simulink model "torqueBalancing2012b"  (Simulink 8.0)
settings: Solver=FixedStepDiscrete  StartTime=0.0  StopTime=CONFIG.SIMULATION_TIME  FixedStep=CONFIG.Ts  RelTol=1e-3
InitFcn:
  | initTorqueBalancing;
values from neighbouring files (symbols this model uses):
  baseToWorldRotationPort = ['/' WBT_modelName '/floatingBaseRotationMatrix:i']    [initTorqueBalancing.m]
  WBT_modelName = 'matlabTorqueBalancing'    [initTorqueBalancing.m]
undefined symbols (not defined in the file or in its folder): bVectorConstraints, CONFIG, ConstraintsMatrix, DiscIntNeverNeededParam, gain, impedencesSat, reg, ROBOT_DOF, ROBOT_DOF_FOR_SIMULINK, sat, SM, sm, Ts
libraries: WBToolboxLibrary x139, simulink x11, WBCLibrary x2
(part 3 of 3)

== matlab function DesValues/State Machine/nu/MATLAB Function ==
  data: JcLeftFoot input double; JcRightFoot input double; activeFeetConstraints input double; y output double; qD input double; reg parameter double
function y = fcn(JcLeftFoot,JcRightFoot,activeFeetConstraints,qD,reg)
%#codegen

Jc = [activeFeetConstraints(1)*JcLeftFoot;
      activeFeetConstraints(2)*JcRightFoot];

pinvJb = (Jc(:,1:6)'*Jc(:,1:6) + reg.pinvDampVb*eye(6))\Jc(:,1:6)';  
  
% pinvJb = pinv(Jc(:,1:6));

y = -pinvJb*Jc(:,7:end)*qD;

== matlab function DesValues/State Machine/stateMachineFCN ==
  data: wrench_rightFoot input double; wrench_leftFoot input double; w_H_b output double; CoMDes output double; qDes output double; constraints output double; state data_store_memory double; CoM_0 input double; q0 input double; l_sole_CoM input double; r_sole_CoM input double; qj input double; t input double; l_sole_H_b input double; r_sole_H_b input double; tSwitch data_store_memory double; sm parameter double; impedances output double; gain parameter double; currentState output double; w_H_r_sole_switch data_store_memory double
function [w_H_b, CoMDes,qDes,constraints,impedances,currentState] = ...
    stateMachineFCN(wrench_rightFoot,wrench_leftFoot,CoM_0, q0, l_sole_CoM,r_sole_CoM,qj, t, l_sole_H_b, r_sole_H_b, sm,gain)
%#codegen
 
[CoMDes,qDes,constraints, currentState,impedances,w_H_b] = ...
    stateMachine(CoM_0, q0, l_sole_CoM,r_sole_CoM,qj, t, wrench_rightFoot,wrench_leftFoot,l_sole_H_b, r_sole_H_b, sm,gain);

== matlab function DesValues/nonlinearImpedances/nonlinearPosturalGains  ==
  data: qDes input double; nonlinearImpedences output double; q input double; qMin input double; qMax input double; gain parameter double
function nonlinearImpedences = fcn(qDes,q,qMin,qMax,gain)
    %#codegen
    impedences_at_0     = gain.impedances;
    increasingRatesImp  = (gain.increasingRatesImp)';
    qTildeMax           = gain.qTildeMax;

    tp =  pi./(2*(qMax-qDes));
    tn = -pi./(2*(qMin-qDes));

    
    qTilde = q - qDes;
            
    nonlinearImpedences = (impedences_at_0'   + increasingRatesImp.*tan(pi.*qTilde./(2*qTildeMax)).^2)';
%                                                increasingRatesImp.*tan((tp.*stepFcn(qTilde) + tn.*stepFcn(-qTilde)).*qTilde).^2)';
                                           
end

function y = stepFcn(x) 
   %#codegen
   y = x > 0; 
end

== matlab function Dump and visualize/plotNorms/norm ==
  data: u input double; normU output double
function normU = fcn(u)
%#codegen

normU = norm(u);

== matlab function Dump and visualize/plotNorms/norm1 ==
  data: u input double; normU output double
function normU = fcn(u)
%#codegen

normU = norm(u);

== matlab function controller_QP/tau(f)  ==
  data: tauModel output double; Sigma output double; NA output double; fHdotDesC1C2 output double; HessianMatrixQP1Foot output double; gradientQP1Foot output double; ConstraintsMatrixQP1Foot output double; bVectorConstraintsQp1Foot output double; HessianMatrixQP2Feet output double; gradientQP2Feet output double; ConstraintsMatrixQP2Feet output double; bVectorConstraintsQp2Feet output double; constraints input double; ROBOT_DOF_FOR_SIMULINK input double; ConstraintsMatrix input double; bVectorConstraints input double; q input double; qDes input double; v input double; M input double; h input double; H input double; w_H_l_sole input double; w_H_r_sole input double; JL input double; JR input double; dJLv input double; dJRv input double; xcom input double; J_CoM input double; desired_x_dx_ddx_CoM input double; impedances input double; intErrorCoM input double; ki_int_qtilde input double; reg parameter double; gain parameter double; errorCoM output double; qTilde output double; f output double; Deltaphi input double
function [tauModel,Sigma,NA,fHdotDesC1C2, ...
          HessianMatrixQP1Foot,gradientQP1Foot,ConstraintsMatrixQP1Foot,bVectorConstraintsQp1Foot,...
          HessianMatrixQP2Feet,gradientQP2Feet,ConstraintsMatrixQP2Feet,bVectorConstraintsQp2Feet,...
          errorCoM,qTilde,f]    =  ...
          controllerFCN(constraints,ROBOT_DOF_FOR_SIMULINK,ConstraintsMatrix,bVectorConstraints,...
          q,qDes,v, M, h , H,w_H_l_sole, w_H_r_sole, JL,JR, dJLv,dJRv, xcom,J_CoM, desired_x_dx_ddx_CoM,...
          impedances, intErrorCoM,ki_int_qtilde,reg,gain,Deltaphi)
%#codegen
pos_leftFoot   = w_H_l_sole(1:3,4);
rotMatLeftFoot = w_H_l_sole(1:3,1:3);

pos_rightFoot   = w_H_r_sole(1:3,4);
rotMatRightFoot = w_H_r_sole(1:3,1:3);

footSize       = gain.footSize;
gainsPCOM      = gain.PCOM;
gainsICOM      = gain.ICOM;
gainsDCOM      = gain.DCOM;
DgainMomentum  = gain.DAngularMomentum;
PgainMomentum  = gain.PAngularMomentum;
dampings       = gain.dampings;

e1              = [1;0;0];
e2              = [0;1;0];
e3              = [0;0;1]; 
ROBOT_DOF       = size(ROBOT_DOF_FOR_SIMULINK,1);


gravAcc         = 9.81;
m               = M(1,1);
Mb              = M(1:6,1:6);
Mbj             = M(1:6,7:end);
% Mj              = M(7:end,7:end);

St              = [  zeros(6,ROBOT_DOF);
                   eye(ROBOT_DOF,ROBOT_DOF)];
grav            = [ zeros(2,1);
                   -m*gravAcc;
                    zeros(3,1)];
                



xDcom           = J_CoM(1:3,:)*v;
qD              = v(7:end);
xDDcomStar      = desired_x_dx_ddx_CoM(:,3) - gainsPCOM*(xcom - desired_x_dx_ddx_CoM(:,1)) - gainsICOM*intErrorCoM - gainsDCOM*(xDcom - desired_x_dx_ddx_CoM(:,2));
Pr              = pos_rightFoot - xcom; % Application point of the contact force on the right foot w.r.t. CoM
Pl              = pos_leftFoot  - xcom; % Application point of the contact force on the left foot w.r.t. CoM


AL = [ eye(3),   zeros(3);
       Sf(Pl),  eye(3)];
AR = [ eye(3), zeros(3);
        Sf(Pr), eye(3) ];
    
A    = [ AL, AR];

Jc   = [ JL*constraints(1) ;
         JR*constraints(2)];
JcDv = [ dJLv*constraints(1) ;
         dJRv*constraints(2)];

JcMinv          = Jc/M;
JcMinvSt        = JcMinv*St;
JcMinvJct       = JcMinv*transpose(Jc);

pinvA         = pinv( A, reg.pinvTol)*constraints(1)*constraints(2) + [inv(AL);zeros(6)]*constraints(1)*(1-constraints(2)) + [zeros(6);inv(AR)]*constraints(2)*(1-constraints(1)); 
% PInv_JcMinvSt = pinv( JcMinvSt, PINV_TOL);
PInv_JcMinvSt = JcMinvSt'/(JcMinvSt*JcMinvSt' + reg.pinvDamp*eye(size(JcMinvSt,1)));
  
% linear approssimation of centroidal orientation
qTilde           =  q-qDes;

HDotDes  = [ m*xDDcomStar ;
            -DgainMomentum*H(4:end)-PgainMomentum*Deltaphi]; 
         
%%%%
        
NL        = eye(ROBOT_DOF) - PInv_JcMinvSt*JcMinvSt;

f_HDot           = pinvA*(HDotDes - grav);

fHdotDesC1C2     =  f_HDot*constraints(1)*constraints(2);

NA               = (eye(12,12)-pinvA*A)*constraints(1)*constraints(2);
JBar             = transpose(Jc(:,7:end)) - Mbj'/Mb*transpose(Jc(:,1:6)); % multiplier of f in tau0

Sigma            = -(PInv_JcMinvSt*JcMinvJct + NL*JBar);
SigmaNA          = Sigma*NA;

tauModel         = PInv_JcMinvSt*(JcMinv*h - JcDv) + NL*(h(7:end) - Mbj'/Mb*h(1:6) - diag(impedances)*qTilde  -ki_int_qtilde -diag(dampings)*NL*qD);

CL               = ConstraintsMatrix; 
CL(end-4,1:3)    = -e3'*rotMatLeftFoot;                
CL(end-3,:)      = [ footSize(1,1)*e3'*rotMatLeftFoot', e2'*rotMatLeftFoot'];
CL(end-2,:)      = [-footSize(1,2)*e3'*rotMatLeftFoot',-e2'*rotMatLeftFoot'];

CL(end-1,:)      = [ footSize(2,1)*e3'*rotMatLeftFoot',-e1'*rotMatLeftFoot'];
CL(end  ,:)      = [-footSize(2,2)*e3'*rotMatLeftFoot', e1'*rotMatLeftFoot'];

CR               = ConstraintsMatrix;
CR(end-4,1:3)    = -e3'*rotMatRightFoot;  
CR(end-3,:)      = [ footSize(1,1)*e3'*rotMatRightFoot', e2'*rotMatRightFoot'];
CR(end-2,:)      = [-footSize(1,2)*e3'*rotMatRightFoot',-e2'*rotMatRightFoot'];

CR(end-1,:)      = [ footSize(2,1)*e3'*rotMatRightFoot',-e1'*rotMatRightFoot'];
CR(end  ,:)      = [-footSize(2,2)*e3'*rotMatRightFoot', e1'*rotMatRightFoot'];


ConstraintsMatrix2Feet    = blkdiag(CL,CR);
bVectorConstraints2Feet   = [bVectorConstraints;bVectorConstraints];

ConstraintsMatrixQP1Foot  = constraints(1) * (1 - constraints(2)) * CL + ...
                           constraints(2) * (1 - constraints(1)) * CR;
bVectorConstraintsQp1Foot = bVectorConstraints;

ConstraintsMatrixQP2Feet  = ConstraintsMatrix2Feet*NA;
bVectorConstraintsQp2Feet = bVectorConstraints2Feet-ConstraintsMatrix2Feet*f_HDot;

HessianMatrixQP2Feet      = SigmaNA'*SigmaNA + eye(size(SigmaNA,2))*reg.HessianQP;
gradientQP2Feet           = SigmaNA'*(tauModel + Sigma*f_HDot);

A1Foot                    = AL*constraints(1)*(1-constraints(2)) + AR*constraints(2)*(1-constraints(1));
HessianMatrixQP1Foot      = A1Foot'*A1Foot + eye(size(A1Foot,2))*reg.HessianQP;
gradientQP1Foot           = -A1Foot'*(HDotDes - grav);

f0                        = -pinv(SigmaNA, reg.pinvTol)*(tauModel + Sigma*f_HDot);

f                         = f_HDot + NA*f0;

errorCoM = xcom - desired_x_dx_ddx_CoM(:,1);

== matlab function emergency stop: joint limits/MATLAB Function ==
  data: umin input double; umax input double; u input double; inRange output double; tol input double
function inRange = checkRange(umin, umax, u, tol)
%#codegen

res = u < umin + tol | u > umax - tol;
res = sum(res);
if res==0
    inRange = 1;
else
    inRange = 0;
    u < umin + tol | u > umax - tol
end

== matlab function DesValues/State Machine Walking/w_H_root_link3/fromImuToHomogeousTransformFCN ==
  data: imu_H_link input double; imu_H_link_0 input double; link_H_root input double; inertial_0 input double; inertial input double; w_H_root output double; CONFIG parameter double
function w_H_root = fromBaseToWorldWithImuFCN(imu_H_link,imu_H_link_0,link_H_root,inertial_0,inertial,CONFIG)
%#codegen
w_H_root = fromBaseToWorldWithImu(imu_H_link,imu_H_link_0,link_H_root,inertial_0,inertial,CONFIG);

== matlab function DesValues/centroidalOrient_partialDer/Jw0_base/Generate_Jw0base/MATLAB Function ==
  data: vb1 output double; vb2 output double; vb3 output double; vb4 output double; vb5 output double; vb6 output double
function [vb1,vb2, vb3, vb4, vb5, vb6] = gen_vb()
%#codegen

vb1 = [1;0;0;0;0;0];
vb2 = [0;1;0;0;0;0];
vb3 = [0;0;1;0;0;0];
vb4 = [0;0;0;1;0;0];
vb5 = [0;0;0;0;1;0];
vb6 = [0;0;0;0;0;1];

end

== matlab function DesValues/centroidalOrient_partialDer/Jw0_base/Generate_Jw0base/MATLAB Function1 ==
  data: H1 input double; Jw0b output double; H2 input double; H3 input double; H4 input double; H5 input double; H6 input double
function Jw0b = reorder_Jwb(H1,H2,H3,H4,H5,H6)
%#codegen

Jw0b = [H1 H2 H3 H4 H5 H6];

end

== matlab function DesValues/centroidalOrient_partialDer/Jc0/MATLAB Function ==
  data: Jclf input double; Jc0 output double; Jcrf input double
function Jc0 = fcn(Jclf,Jcrf)
%#codegen

Jc0 = [Jclf;Jcrf];

end

== matlab function DesValues/centroidalOrient_partialDer/Jw0_joints/Generate_Jw0torso/MATLAB Function ==
  data: dqj1 output double; dqj2 output double; dqj3 output double
function [dqj1,dqj2,dqj3] = gen_vb()
%#codegen
ndof = 23;

dqj1 = zeros(ndof,1);
dqj2 = zeros(ndof,1);
dqj3 = zeros(ndof,1);

dqj1(1) = 1;
dqj2(2) = 1;
dqj3(3) = 1;

end

== matlab function DesValues/centroidalOrient_partialDer/Jw0_joints/Generate_Jw0torso/MATLAB Function1 ==
  data: H1 input double; Jw0j1 output double; H2 input double; H3 input double
function Jw0j1 = reorder_Jwj(H1,H2,H3)
%#codegen

Jw0j1 = [H1 H2 H3];

end

== matlab function DesValues/centroidalOrient_partialDer/Jw0_joints/Generate_Jw0Rarm/MATLAB Function ==
  data: dqj9 output double; dqj10 output double; dqj11 output double; dqj12 output double; dqj13 output double
function [dqj9,dqj10, dqj11, dqj12, dqj13] = gen_vb()
%#codegen
ndof = 23;

dqj9  = zeros(ndof,1);
dqj10 = dqj9;
dqj11 = dqj10;
dqj12 = dqj11;
dqj13 = dqj12;

dqj9(9)  = 1;
dqj10(10) = 1;
dqj11(11) = 1;
dqj12(12) = 1;
dqj13(13) = 1;

end

== matlab function DesValues/centroidalOrient_partialDer/Jw0_joints/Generate_Jw0Rarm/MATLAB Function1 ==
  data: H1 input double; Jw0j3 output double; H2 input double; H3 input double; H4 input double; H5 input double
function Jw0j3 = reorder_Jwj(H1,H2,H3,H4,H5)
%#codegen

Jw0j3 = [H1 H2 H3 H4 H5];

end

== matlab function DesValues/centroidalOrient_partialDer/Jw0_joints/Generate_Jw0Lleg/MATLAB Function ==
  data: dqj14 output double; dqj15 output double; dqj16 output double; dqj17 output double; dqj18 output double
function [dqj14,dqj15, dqj16, dqj17, dqj18] = gen_vb()
%#codegen
ndof = 23;

dqj14 = zeros(ndof,1);
dqj15 = dqj14;
dqj16 = dqj15;
dqj17 = dqj16;
dqj18 = dqj17;

dqj14(14) = 1;
dqj15(15) = 1;
dqj16(16) = 1;
dqj17(17) = 1;
dqj18(18) = 1;

end

== matlab function DesValues/centroidalOrient_partialDer/Jw0_joints/Generate_Jw0Lleg/MATLAB Function1 ==
  data: H1 input double; Jw0j4 output double; H2 input double; H3 input double; H4 input double; H5 input double
function Jw0j4 = reorder_Jwj(H1,H2,H3,H4,H5)
%#codegen

Jw0j4 = [H1 H2 H3 H4 H5];

end

== matlab function DesValues/centroidalOrient_partialDer/Jw0_joints/Generate_Jw0Rleg/MATLAB Function ==
  data: dqj19 output double; dqj20 output double; dqj21 output double; dqj22 output double; dqj23 output double
function [dqj19,dqj20, dqj21, dqj22, dqj23] = gen_vb()
%#codegen
ndof = 23;

dqj19 = zeros(ndof,1);
dqj20 = dqj19;
dqj21 = dqj20;
dqj22 = dqj21;
dqj23 = dqj22;

dqj19(19) = 1;
dqj20(20) = 1;
dqj21(21) = 1;
dqj22(22) = 1;
dqj23(23) = 1;

end

== matlab function DesValues/centroidalOrient_partialDer/Jw0_joints/Generate_Jw0Rleg/MATLAB Function1 ==
  data: H1 input double; Jw0j5 output double; H2 input double; H3 input double; H4 input double; H5 input double
function Jw0j5 = reorder_Jwj(H1,H2,H3,H4,H5)
%#codegen

Jw0j5 = [H1 H2 H3 H4 H5];

end

== matlab function DesValues/centroidalOrient_partialDer/Jw0_joints/MATLAB Function ==
  data: Jw01 input double; Jw0j output double; Jw02 input double; Jw03 input double; Jw04 input double; Jw05 input double
function Jw0j = fcn(Jw01,Jw02,Jw03,Jw04,Jw05)
%#codegen

Jw0j = [Jw01 Jw02 Jw03 Jw04 Jw05];

== matlab function DesValues/centroidalOrient_partialDer_at_0/MATLAB Function ==
  data: Jclf input double; vbar output double; Deltaqj input double
function vbar  = GeneratevectorsForH(Jclf,Deltaqj)
%#codegen

vbar  = -(eye(6)/Jclf(1:6,1:6))*Jclf(1:6,7:end)*Deltaqj;

end

== matlab function DesValues/centroidalOrient_partialDer/Jw0_joints/Generate_Jw0Larm/MATLAB Function ==
  data: dqj4 output double; dqj5 output double; dqj6 output double; dqj7 output double; dqj8 output double
function [dqj4,dqj5, dqj6, dqj7, dqj8] = gen_vb()
%#codegen
ndof = 23;

dqj4 = zeros(ndof,1);
dqj5 = dqj4;
dqj6 = dqj5;
dqj7 = dqj6;
dqj8 = dqj7;

dqj4(4) = 1;
dqj5(5) = 1;
dqj6(6) = 1;
dqj7(7) = 1;
dqj8(8) = 1;

end

== matlab function DesValues/centroidalOrient_partialDer/Jw0_joints/Generate_Jw0Larm/MATLAB Function1 ==
  data: H1 input double; Jw0j2 output double; H2 input double; H3 input double; H4 input double; H5 input double
function Jw0j2 = reorder_Jwj(H1,H2,H3,H4,H5)
%#codegen

Jw0j2 = [H1 H2 H3 H4 H5];

end
